simulink model "deadMansSwitch_tester"  (R2016a)
settings: Solver=FixedStepAuto  StartTime=0.0  StopTime=5  FixedStep=0.01  RelTol=1e-3
settings Model: Creator=sprinkle  LastModifiedBy=sprinkle

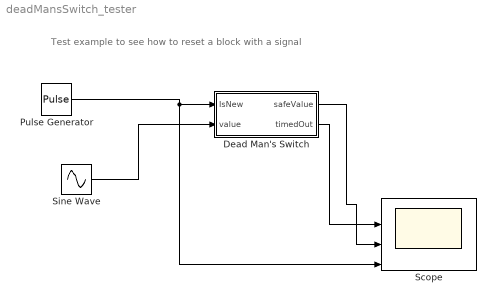
== system deadMansSwitch_tester ==
  note: Test example to see how to reset a block with a signal
  Dead Man's Switch : Subsystem  TreatAsAtomicUnit=on  mask{stepSize=0.01, timeout=0.2}
      mask prompts: stepSize "Simulation step size"; timeout "Timeout (in seconds)"
  Pulse Generator : DiscretePulseGenerator  PulseType=Time based  Period=1  PulseWidth=35
  Scope : Scope  NumInputPorts=4
  Sine Wave : Sin  SampleTime=0
  wires:
  Pulse Generator/1 -> Dead Man's Switch/1(IsNew), Scope/4
  Sine Wave/1 -> Dead Man's Switch/2(value)
  Dead Man's Switch/1(safeValue) -> Scope/3
  Dead Man's Switch/2(timedOut) -> Scope/2

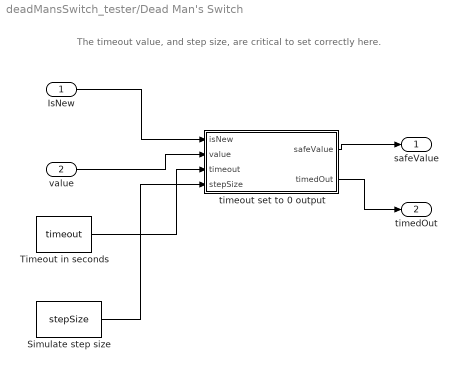
== system deadMansSwitch_tester/Dead Man's Switch ==
  note: The timeout value, and step size, are critical to set correctly here.
  IsNew : Inport
  value : Inport  Port=2
  Simulate step size : Constant  Value=stepSize
  Timeout in seconds : Constant  Value=timeout
  timeout set to 0 output : MATLAB Function  TreatAsAtomicUnit=on
  safeValue : Outport  InitialOutput=[0]
  timedOut : Outport  Port=2  InitialOutput=[0]
  wires:
  IsNew/1 -> timeout set to 0 output/1(isNew)
  timeout set to 0 output/1(safeValue) -> safeValue/1
  value/1 -> timeout set to 0 output/2(value)
  Timeout in seconds/1 -> timeout set to 0 output/3(timeout)
  timeout set to 0 output/2(timedOut) -> timedOut/1
  Simulate step size/1 -> timeout set to 0 output/4(stepSize)

== matlab function deadMansSwitch_tester/Dead Man's Switch/timeout set to 0 output ==
  data: isNew input; safeValue output; value input; timeout input; timedOut output; stepSize input
function [safeValue,timedOut] = fcn(isNew,value,timeout,stepSize)
%#codegen
persistent sinceLastMsg
timedOut=true;
if isempty(sinceLastMsg)
    sinceLastMsg=(timeout/stepSize)+1;
end

safeValue=0;
% if no new message
% after timeout, we output 0
if( isNew == true )
    sinceLastMsg = 0;
else
    sinceLastMsg = sinceLastMsg+1;
end

% Note: we require step size as an input here, and depend on our
% system being executed at a regular rate, or bad things will happen
if( sinceLastMsg < timeout/stepSize )
    timedOut = false;
end
    
if( timedOut == false )
    safeValue = value;
end
